simulink model "MySim3"  (R2014b)
settings: Solver=ode45  StartTime=0.0  StopTime=10.0  RelTol=1e-3
values from neighbouring files (symbols this model uses):
  K = place(A,B,PoleArray)    [script2.m]
settings Model: Creator=el12074  LastModifiedBy=gvavou5

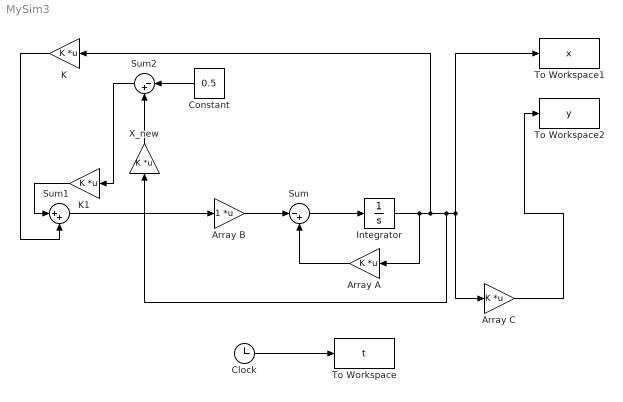
== system MySim3 ==
  Array A : Gain  Gain=K  Multiplication=Matrix(K*u)
  Array B : Gain  Multiplication=Matrix(K*u)
  Array C : Gain  Gain=K  Multiplication=Matrix(K*u)
  Clock : Clock
  Constant : Constant  Value=0.5
  Integrator : Integrator
  Sum : Sum  Inputs=|-+
  Sum1 : Sum  Inputs=|++
  Sum2 : Sum  Inputs=|-+
  To Workspace : ToWorkspace  VariableName=t  SaveFormat=Timeseries  SampleTime=-1
  To Workspace1 : ToWorkspace  VariableName=x  SaveFormat=Timeseries  SampleTime=-1
  To Workspace2 : ToWorkspace  VariableName=y  SaveFormat=Timeseries  SampleTime=-1
  X_new : Gain  Gain=K  Multiplication=Matrix(K*u)
  Κ : Gain  Gain=K  Multiplication=Matrix(K*u)
  Κ1 : Gain  Gain=K  Multiplication=Matrix(K*u)
  wires:
  Array B/1 -> Sum/1
  Array A/1 -> Sum/2
  Sum/1 -> Integrator/1
  Array C/1 -> To Workspace2/1
  Clock/1 -> To Workspace/1
  Sum1/1 -> Array B/1
  Constant/1 -> Sum2/1
  X_new/1 -> Sum2/2
  Sum2/1 -> Κ1/1
  Κ1/1 -> Sum1/1
  Κ/1 -> Sum1/2
  Integrator/1 -> X_new/1, To Workspace1/1, Array C/1, Κ/1, Array A/1
